simulink model "Balance"  (R2020a)
settings: Solver=FixedStepDiscrete  StartTime=0.0  StopTime=10.0  FixedStep=0.001  RelTol=1e-3
libraries: TIMERS_Lib x5, GPIO_Lib x4, USART_Lib x1, STM32_Config_Lib x1
settings Model: Creator=xiang  LastModifiedBy=Administrator
settings OptimizationCC: DefaultParameterBehavior=Inlined  EnhancedBackFolding=on  PassReuseOutputArgsAs=Individual arguments  ZeroExternalMemoryAtStartup=off  ZeroInternalMemoryAtStartup=off  OptimizeBlockOrder=speed  DifferentSizesBufferReuse=on  OptimizationCustomize=off  EfficientTunableParamExpr=on
settings DebuggingCC: MultiTaskDSMMsg=none  ParameterTunabilityLossMsg=error
settings HardwareCC: ProdBitPerPointer=32  ProdBitPerSizeT=32  ProdBitPerPtrDiffT=32  ProdLargestAtomicInteger=Long  ProdWordSize=32  ProdHWDeviceType=STM32CortexM
settings SFSimCC: SimCustomHeaderCode="#include \"myfile.h\""  SimUserSources="\"D:\\BMS\\CubeMx\\CubeMx_0804\\XSZ20210804\\myfile.c\""  MATLABDynamicMemAlloc=off
settings RTWCC: Description=stm32 (Embedded Target)  SystemTargetFile=stm32.tlc  TemplateMakefile=stm32.tmf  GenerateReport=on  RTWUseSimCustomCode=on  CustomHeaderCode="#include \"myfile.h\""  CustomSource="\"D:\\BMS\\CubeMx\\CubeMx_0804\\XSZ20210804\\myfile.c\""
settings CodeAppCC: ForceParamTrailComments=on  IgnoreCustomStorageClasses=off  MaxIdLength=64  OperatorAnnotations=on  SimulinkDataObjDesc=on  SFDataObjDesc=on  CustomSymbolStrType=$N$R$M  SimulinkBlockComments=off
settings STFCustomTargetCC: TargetLangStandard=C99 (ISO)  CodeReplacementLibrary=ARM CMSIS SIN COS  MultiwordLength=256  ParMdlRefBuildCompliant=on  IncludeMdlTerminateFcn=off  CombineOutputUpdateFcns=on  ERTCustomFileBanners=on  SupportContinuousTime=off  SupportNonInlinedSFcns=off  RemoveResetFunc=on  MATLABClassNameForMDSCustomization=Simulink.SoftwareTarget.ERTCustomization  SystemTargetFile=stm32.tlc
settings ERTTargetCC: TargetLangStandard=C99 (ISO)  CodeReplacementLibrary=ARM CMSIS SIN COS  CompOptLevelCompliant=off  ConcurrentExecutionCompliant=off  IncludeMdlTerminateFcn=off  ModelStepFunctionPrototypeControlCompliant=off  CPPClassGenCompliant=off  UseToolchainInfoCompliant=off  ExtModeStaticAllocSize=256  ExtModeMexFile=ext_serial_win32_comm  ExtModeMexArgs=0,1,115200,10  InlinedParameterPlacement=NonHierarchical  ERTSrcFileBannerTemplate=sourceFileTemplate.cgt  ERTHdrFileBannerTemplate=sourceFileTemplate.cgt  ERTDataSrcFileTemplate=sourceFileTemplate.cgt  ERTDataHdrFileTemplate=sourceFileTemplate.cgt  ERTCustomFileTemplate=customRoutineProcess.tlc

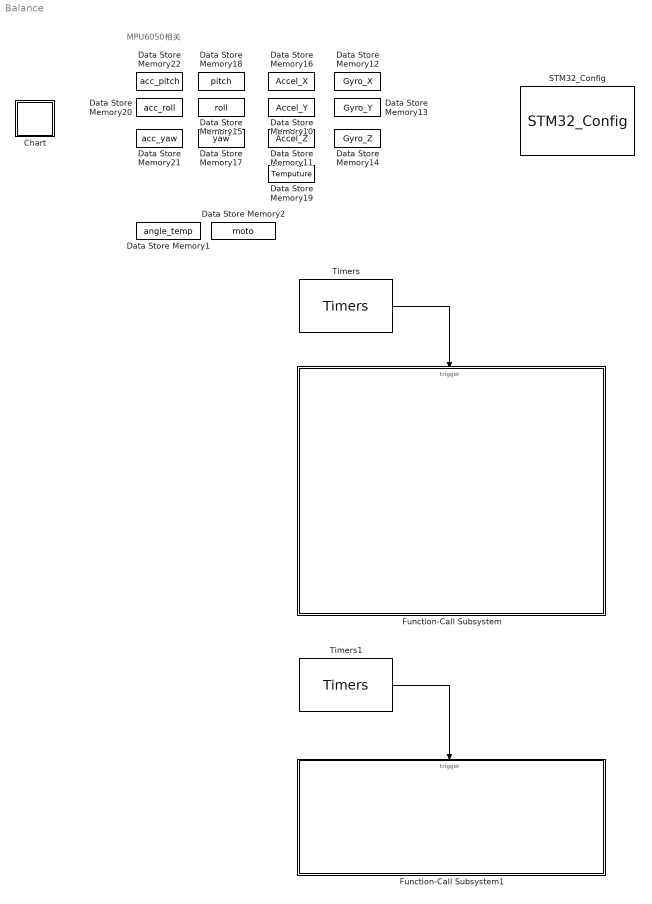
== system Balance ==
  note: MPU6050相关
  Chart : Stateflow chart  Priority=1  TreatAsAtomicUnit=on
  Data Store Memory1 : DataStoreMemory  DataStoreName=angle_temp  ReadBeforeWriteMsg=warning  WriteAfterWriteMsg=warning  WriteAfterReadMsg=warning  ShowAdditionalParam=off  OutDataTypeStr=single
      settings: RTWStateStorageClass=ExportedGlobal
  Data Store Memory10 : DataStoreMemory  DataStoreName=Accel_Y  ReadBeforeWriteMsg=warning  WriteAfterWriteMsg=warning  WriteAfterReadMsg=warning  ShowAdditionalParam=off  OutDataTypeStr=double
      settings: RTWStateStorageClass=ExportedGlobal
  Data Store Memory11 : DataStoreMemory  DataStoreName=Accel_Z  ReadBeforeWriteMsg=warning  WriteAfterWriteMsg=warning  WriteAfterReadMsg=warning  ShowAdditionalParam=off  OutDataTypeStr=double
      settings: RTWStateStorageClass=ExportedGlobal
  Data Store Memory12 : DataStoreMemory  DataStoreName=Gyro_X  ReadBeforeWriteMsg=warning  WriteAfterWriteMsg=warning  WriteAfterReadMsg=warning  ShowAdditionalParam=off  OutDataTypeStr=double
      settings: RTWStateStorageClass=ExportedGlobal
  Data Store Memory13 : DataStoreMemory  DataStoreName=Gyro_Y  ReadBeforeWriteMsg=warning  WriteAfterWriteMsg=warning  WriteAfterReadMsg=warning  ShowAdditionalParam=off  OutDataTypeStr=double
      settings: RTWStateStorageClass=ExportedGlobal
  Data Store Memory14 : DataStoreMemory  DataStoreName=Gyro_Z  ReadBeforeWriteMsg=warning  WriteAfterWriteMsg=warning  WriteAfterReadMsg=warning  ShowAdditionalParam=off  OutDataTypeStr=double
      settings: RTWStateStorageClass=ExportedGlobal
  Data Store Memory15 : DataStoreMemory  DataStoreName=roll  ReadBeforeWriteMsg=warning  WriteAfterWriteMsg=warning  WriteAfterReadMsg=warning  ShowAdditionalParam=off  OutDataTypeStr=double
      settings: RTWStateStorageClass=ExportedGlobal
  Data Store Memory16 : DataStoreMemory  DataStoreName=Accel_X  ReadBeforeWriteMsg=warning  WriteAfterWriteMsg=warning  WriteAfterReadMsg=warning  ShowAdditionalParam=off  OutDataTypeStr=double
      settings: RTWStateStorageClass=ExportedGlobal
  Data Store Memory17 : DataStoreMemory  DataStoreName=yaw  ReadBeforeWriteMsg=warning  WriteAfterWriteMsg=warning  WriteAfterReadMsg=warning  ShowAdditionalParam=off  OutDataTypeStr=double
      settings: RTWStateStorageClass=ExportedGlobal
  Data Store Memory18 : DataStoreMemory  DataStoreName=pitch  ReadBeforeWriteMsg=warning  WriteAfterWriteMsg=warning  WriteAfterReadMsg=warning  ShowAdditionalParam=off  OutDataTypeStr=double
      settings: RTWStateStorageClass=ExportedGlobal
  Data Store Memory19 : DataStoreMemory  DataStoreName=Temputure  ReadBeforeWriteMsg=warning  WriteAfterWriteMsg=warning  WriteAfterReadMsg=warning  ShowAdditionalParam=off  OutDataTypeStr=double
      settings: RTWStateStorageClass=ExportedGlobal
  Data Store Memory2 : DataStoreMemory  DataStoreName=moto  ReadBeforeWriteMsg=warning  WriteAfterWriteMsg=warning  WriteAfterReadMsg=warning  ShowAdditionalParam=off  OutDataTypeStr=double
      settings: RTWStateStorageClass=ExportedGlobal
  Data Store Memory20 : DataStoreMemory  DataStoreName=acc_roll  ReadBeforeWriteMsg=warning  WriteAfterWriteMsg=warning  WriteAfterReadMsg=warning  ShowAdditionalParam=off  OutDataTypeStr=double
      settings: RTWStateStorageClass=ExportedGlobal
  Data Store Memory21 : DataStoreMemory  DataStoreName=acc_yaw  ReadBeforeWriteMsg=warning  WriteAfterWriteMsg=warning  WriteAfterReadMsg=warning  ShowAdditionalParam=off  OutDataTypeStr=double
      settings: RTWStateStorageClass=ExportedGlobal
  Data Store Memory22 : DataStoreMemory  DataStoreName=acc_pitch  ReadBeforeWriteMsg=warning  WriteAfterWriteMsg=warning  WriteAfterReadMsg=warning  ShowAdditionalParam=off  OutDataTypeStr=double
      settings: RTWStateStorageClass=ExportedGlobal
  Function-Call Subsystem : Subsystem  TreatAsAtomicUnit=on
  Function-Call Subsystem1 : Subsystem  TreatAsAtomicUnit=on
  STM32_Config : STM32_Config_Lib/STM32_Config  Priority=0  Project_Path=.\  Config_File=XSZ20210804.ioc  MCU_Name=STM32F103VETx
      settings: SourceProductName=Target Support Package - STM32 Adapter
  Timers : TIMERS_Lib/Timers  currentTIM=TIM1  TIM_Name=TIM1  sysUsingTimer=off  TIM_APBClock=72000000  TIM_Set_Clk=off  TIM_Prescaler=7199  TIM_Clock=10000.00  Variable_frequency=off  TIM_Set_OutFreq=on  TIM_ARR=50  Output_frequency=200.00  Repetition_counter=0  TIM_Mode=Up  TIM_DMA=none  TIM_IRQ=off  TIM_IRQ_ONLY=on  TIM_UP=on  TIM_TRG=off  TIM_COM=off  TIM_BRK=off  NbTIM=3  CH1_enable=off  CH1N_enable=off  CH1_type=Unknown  CH1_DMA=off  CH1_int=off  CH1_edge=Rising  CH1_div=1  CH1_variable_duty=off  CH1_set_pulse=off  CH1_output_duty=0.00  CH1_pulse=0  CH2_enable=off  CH2N_enable=off  CH2_type=Unknown  CH2_DMA=off  CH2_int=off  CH2_edge=Rising  CH2_div=1  CH2_variable_duty=off  CH2_set_pulse=off  CH2_output_duty=0.00  CH2_pulse=0  CH3_enable=off  CH3N_enable=off  CH3_type=Unknown  CH3_DMA=off  CH3_int=off  CH3_edge=Rising  CH3_div=1  CH3_variable_duty=off  CH3_set_pulse=off  CH3_output_duty=0.00  CH3_pulse=0  CH4_enable=off  CH4N_enable=off  CH4_type=Unknown  CH4_DMA=off  CH4_int=off  CH4_edge=Rising  CH4_div=1  CH4_variable_duty=off  CH4_set_pulse=off  CH4_output_duty=0.00  CH4_pulse=0
      settings: SourceProductName=Target Support Package - STM32 Adapter
  Timers1 : TIMERS_Lib/Timers  currentTIM=TIM3  TIM_Name=TIM3  sysUsingTimer=off  TIM_APBClock=72000000  TIM_Set_Clk=off  TIM_Prescaler=7199  TIM_Clock=10000.00  Variable_frequency=off  TIM_Set_OutFreq=off  TIM_ARR=1000  Output_frequency=10.00  Repetition_counter=0  TIM_Mode=Up  TIM_DMA=none  TIM_IRQ=on  TIM_IRQ_ONLY=on  TIM_UP=on  TIM_TRG=off  TIM_COM=off  TIM_BRK=off  NbTIM=3  CH1_enable=off  CH1N_enable=off  CH1_type=Unknown  CH1_DMA=off  CH1_int=off  CH1_edge=Rising  CH1_div=1  CH1_variable_duty=off  CH1_set_pulse=off  CH1_output_duty=0.00  CH1_pulse=0  CH2_enable=off  CH2N_enable=off  CH2_type=Unknown  CH2_DMA=off  CH2_int=off  CH2_edge=Rising  CH2_div=1  CH2_variable_duty=off  CH2_set_pulse=off  CH2_output_duty=0.00  CH2_pulse=0  CH3_enable=off  CH3N_enable=off  CH3_type=Unknown  CH3_DMA=off  CH3_int=off  CH3_edge=Rising  CH3_div=1  CH3_variable_duty=off  CH3_set_pulse=off  CH3_output_duty=0.00  CH3_pulse=0  CH4_enable=off  CH4N_enable=off  CH4_type=Unknown  CH4_DMA=off  CH4_int=off  CH4_edge=Rising  CH4_div=1  CH4_variable_duty=off  CH4_set_pulse=off  CH4_output_duty=0.00  CH4_pulse=0
      settings: SourceProductName=Target Support Package - STM32 Adapter
  wires:
  Timers/1 -> Function-Call Subsystem/Trigger
  Timers1/1 -> Function-Call Subsystem1/Trigger

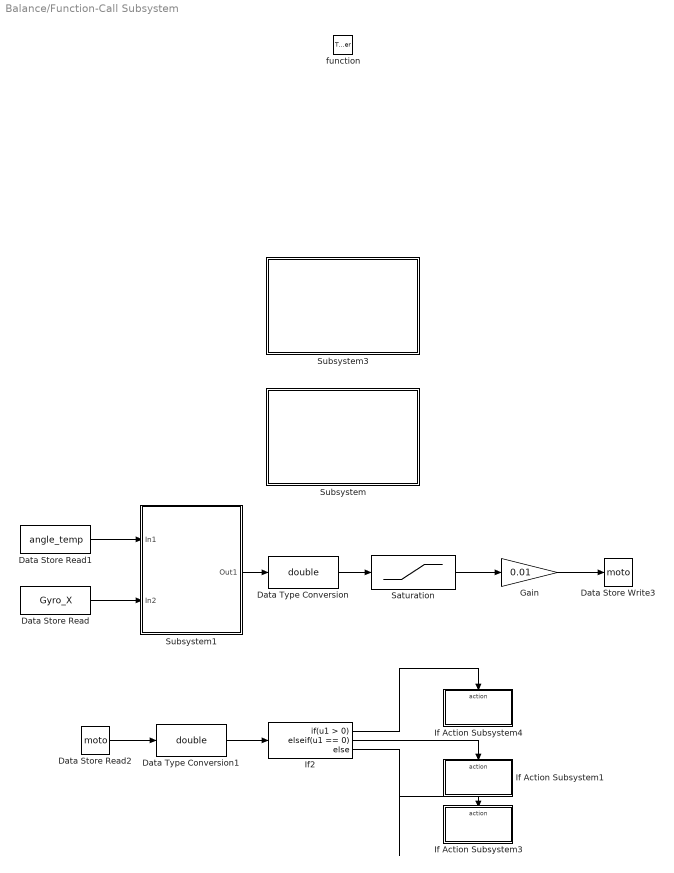
== system Balance/Function-Call Subsystem ==
  function : TriggerPort  TriggerType=function-call  VariantControl=Variant
  Data Store Read : DataStoreRead  DataStoreName=Gyro_X
  Data Store Read1 : DataStoreRead  DataStoreName=angle_temp
  Data Store Read2 : DataStoreRead  DataStoreName=moto
  Data Store Write3 : DataStoreWrite  DataStoreName=moto
  Data Type Conversion : DataTypeConversion  OutDataTypeStr=double
  Data Type Conversion1 : DataTypeConversion  OutDataTypeStr=double
  Gain : Gain  Gain=0.01
  If Action Subsystem1 : Subsystem  TreatAsAtomicUnit=on
  If Action Subsystem3 : Subsystem  TreatAsAtomicUnit=on
  If Action Subsystem4 : Subsystem  TreatAsAtomicUnit=on
  If2 : If  ElseIfExpressions=u1 == 0
  Saturation : Saturate  UpperLimit=1000  LowerLimit=-1000
  Subsystem : Subsystem
  Subsystem1 : Subsystem  Priority=1
  Subsystem3 : Subsystem  Priority=2
  wires:
  If2/1 -> If Action Subsystem4/Action
  If2/2 -> If Action Subsystem1/Action
  If2/3 -> If Action Subsystem3/Action
  Data Store Read1/1 -> Subsystem1/1(In1)
  Data Store Read/1 -> Subsystem1/2(In2)
  Saturation/1 -> Gain/1
  Subsystem1/1(Out1) -> Data Type Conversion/1
  Data Type Conversion/1 -> Saturation/1
  Gain/1 -> Data Store Write3/1
  Data Store Read2/1 -> Data Type Conversion1/1
  Data Type Conversion1/1 -> If2/1

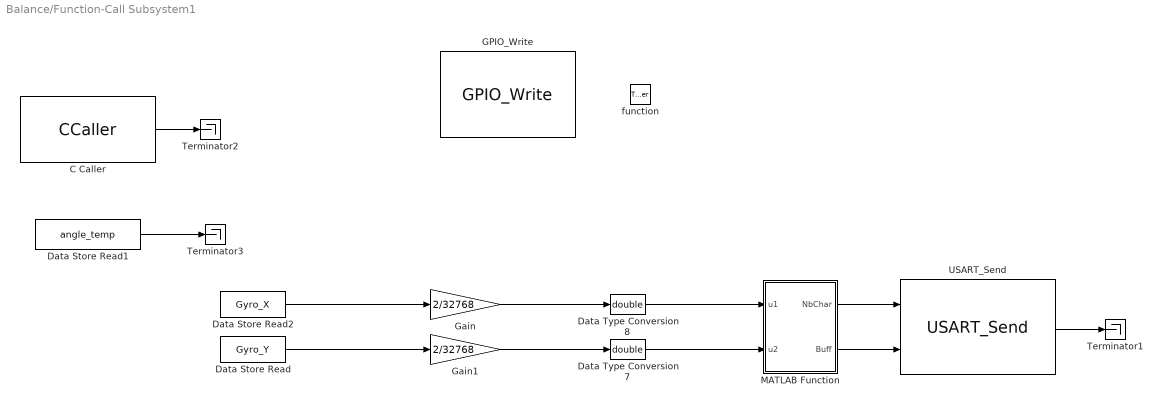
== system Balance/Function-Call Subsystem1 ==
  function : TriggerPort  TriggerType=function-call  VariantControl=Variant
  C Caller : CCaller  FunctionName=Read_Temperature  PortSpecificationStruct="%)30     .    & (   8    (     @         %    \"     $    !     0         %  0 \"0    $    _    07)G3F%M90  4&]R=$YA;64 4V-O<&4     26YD97@     5'EP90      4VEZ90      27-';&]B86P   X    P    !@    @    $          4    (     0    ,    !         !   P!O=70 #@   #     &    \"     0         !0    @    !     P    $         $  # &]U=  .    .     8    (    !          %    \"     $    &     0         0    !@   $]U='!U=   #@   #@    &    \"     8         !0    @    !     0    $         \"0    @               X    X    !@    @    $          4    (     0    4    !         !     %    :6YT,S(    .    ,     8    (    !          %    \"     $    !     0         0  $ ,0    X    P    !@    @    ) @        4    (     0    $    !          (  0"
  Data Store Read : DataStoreRead  DataStoreName=Gyro_Y
  Data Store Read1 : DataStoreRead  DataStoreName=angle_temp
  Data Store Read2 : DataStoreRead  DataStoreName=Gyro_X
  Data Type Conversion7 : DataTypeConversion  OutDataTypeStr=double
  Data Type Conversion8 : DataTypeConversion  OutDataTypeStr=double
  GPIO_Write : GPIO_Lib/GPIO_Write  Port_name=GPIOB  Pin0=on  Toggle_Pin0=on  Pin1=off  Toggle_Pin1=off  Pin2=off  Toggle_Pin2=off  Pin3=off  Toggle_Pin3=off  Pin4=off  Toggle_Pin4=off  Pin5=off  Toggle_Pin5=off  Pin6=off  Toggle_Pin6=off  Pin7=off  Toggle_Pin7=off  Pin8=off  Toggle_Pin8=off  Pin9=off  Toggle_Pin9=off  Pin10=off  Toggle_Pin10=off  Pin11=off  Toggle_Pin11=off  Pin12=off  Toggle_Pin12=off  Pin13=off  Toggle_Pin13=off  Pin14=off  Toggle_Pin14=off  Pin15=off  Toggle_Pin15=off  PinList="GPIOA4  5GPIOB0"
      settings: SourceProductName=Target Support Package - STM32 Adapter
  Gain : Gain  Gain=2/32768
  Gain1 : Gain  Gain=2/32768
  MATLAB Function : MATLAB Function  TreatAsAtomicUnit=on
  Terminator1 : Terminator
  Terminator2 : Terminator
  Terminator3 : Terminator
  USART_Send : USART_Lib/USART_Send  USART_name=USART1  Buff_size=500  nbUsart=1  usartMode=Asynchronous  usartDma_Rx=off  usartDma_Tx=off  usartIt=off
      settings: SourceProductName=Target Support Package - STM32 Adapter
  wires:
  Data Type Conversion8/1 -> MATLAB Function/1(u1)
  Data Type Conversion7/1 -> MATLAB Function/2(u2)
  MATLAB Function/2(Buff) -> USART_Send/2
  USART_Send/1 -> Terminator1/1
  MATLAB Function/1(NbChar) -> USART_Send/1
  C Caller/1 -> Terminator2/1
  Data Store Read1/1 -> Terminator3/1
  Data Store Read2/1 -> Gain/1
  Data Store Read/1 -> Gain1/1
  Gain/1 -> Data Type Conversion8/1
  Gain1/1 -> Data Type Conversion7/1

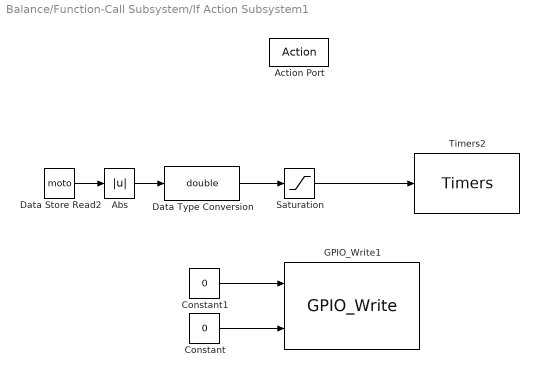
== system Balance/Function-Call Subsystem/If Action Subsystem1 ==
  Action Port : ActionPort  ActionPortLabel=elseif(u1 == 0)
  Abs : Abs
  Constant : Constant  Value=0
  Constant1 : Constant  Value=0
  Data Store Read2 : DataStoreRead  DataStoreName=moto
  Data Type Conversion : DataTypeConversion  OutDataTypeStr=double
  GPIO_Write1 : GPIO_Lib/GPIO_Write  Port_name=GPIOA  Pin0=off  Toggle_Pin0=off  Pin1=off  Toggle_Pin1=off  Pin2=off  Toggle_Pin2=off  Pin3=off  Toggle_Pin3=off  Pin4=on  Toggle_Pin4=off  Pin5=on  Toggle_Pin5=off  Pin6=off  Toggle_Pin6=off  Pin7=off  Toggle_Pin7=off  Pin8=off  Toggle_Pin8=off  Pin9=off  Toggle_Pin9=off  Pin10=off  Toggle_Pin10=off  Pin11=off  Toggle_Pin11=off  Pin12=off  Toggle_Pin12=off  Pin13=off  Toggle_Pin13=off  Pin14=off  Toggle_Pin14=off  Pin15=off  Toggle_Pin15=off  PinList="GPIOA4  5GPIOB0"
      settings: SourceProductName=Target Support Package - STM32 Adapter
  Saturation : Saturate  UpperLimit=100  LowerLimit=0
  Timers2 : TIMERS_Lib/Timers  currentTIM=TIM2  TIM_Name=TIM2  sysUsingTimer=off  TIM_APBClock=72000000  TIM_Set_Clk=off  TIM_Prescaler=71  TIM_Clock=1000000.00  Variable_frequency=off  TIM_Set_OutFreq=off  TIM_ARR=1000  Output_frequency=1000.00  Repetition_counter=0  TIM_Mode=Up  TIM_DMA=none  TIM_IRQ=off  TIM_IRQ_ONLY=off  TIM_UP=off  TIM_TRG=off  TIM_COM=off  TIM_BRK=off  NbTIM=3  CH1_enable=off  CH1N_enable=off  CH1_type=Unknown  CH1_DMA=off  CH1_int=off  CH1_edge=Rising  CH1_div=1  CH1_variable_duty=off  CH1_set_pulse=off  CH1_output_duty=0.00  CH1_pulse=0  CH2_enable=off  CH2N_enable=off  CH2_type=Unknown  CH2_DMA=off  CH2_int=off  CH2_edge=Rising  CH2_div=1  CH2_variable_duty=off  CH2_set_pulse=off  CH2_output_duty=0.00  CH2_pulse=0  CH3_enable=on  CH3N_enable=off  CH3_type=Output_PWM  CH3_DMA=off  CH3_int=off  CH3_edge=Rising  CH3_div=1  CH3_variable_duty=on  CH3_set_pulse=on  CH3_output_duty=80.00  CH3_pulse=800  CH4_enable=off  CH4N_enable=off  CH4_type=Unknown  CH4_DMA=off  CH4_int=off  CH4_edge=Rising  CH4_div=1  CH4_variable_duty=off  CH4_set_pulse=off  CH4_output_duty=0.00  CH4_pulse=0
      settings: SourceProductName=Target Support Package - STM32 Adapter
  wires:
  Constant1/1 -> GPIO_Write1/1
  Constant/1 -> GPIO_Write1/2
  Saturation/1 -> Timers2/1
  Data Type Conversion/1 -> Saturation/1
  Data Store Read2/1 -> Abs/1
  Abs/1 -> Data Type Conversion/1

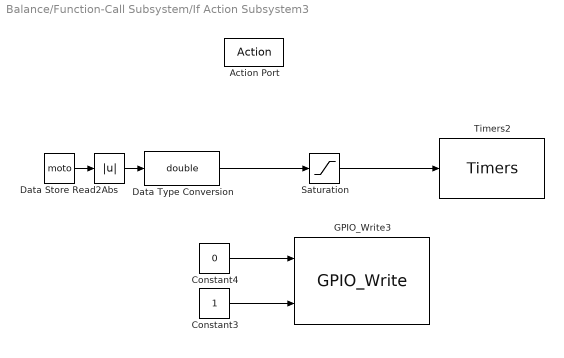
== system Balance/Function-Call Subsystem/If Action Subsystem3 ==
  Action Port : ActionPort  ActionPortLabel=else
  Abs : Abs
  Constant3 : Constant
  Constant4 : Constant  Value=0
  Data Store Read2 : DataStoreRead  DataStoreName=moto
  Data Type Conversion : DataTypeConversion  OutDataTypeStr=double
  GPIO_Write3 : GPIO_Lib/GPIO_Write  Port_name=GPIOA  Pin0=off  Toggle_Pin0=off  Pin1=off  Toggle_Pin1=off  Pin2=off  Toggle_Pin2=off  Pin3=off  Toggle_Pin3=off  Pin4=on  Toggle_Pin4=off  Pin5=on  Toggle_Pin5=off  Pin6=off  Toggle_Pin6=off  Pin7=off  Toggle_Pin7=off  Pin8=off  Toggle_Pin8=off  Pin9=off  Toggle_Pin9=off  Pin10=off  Toggle_Pin10=off  Pin11=off  Toggle_Pin11=off  Pin12=off  Toggle_Pin12=off  Pin13=off  Toggle_Pin13=off  Pin14=off  Toggle_Pin14=off  Pin15=off  Toggle_Pin15=off  PinList="GPIOA4  5GPIOB0"
      settings: SourceProductName=Target Support Package - STM32 Adapter
  Saturation : Saturate  UpperLimit=100  LowerLimit=0
  Timers2 : TIMERS_Lib/Timers  currentTIM=TIM2  TIM_Name=TIM2  sysUsingTimer=off  TIM_APBClock=72000000  TIM_Set_Clk=off  TIM_Prescaler=71  TIM_Clock=1000000.00  Variable_frequency=off  TIM_Set_OutFreq=off  TIM_ARR=1000  Output_frequency=1000.00  Repetition_counter=0  TIM_Mode=Up  TIM_DMA=none  TIM_IRQ=off  TIM_IRQ_ONLY=off  TIM_UP=off  TIM_TRG=off  TIM_COM=off  TIM_BRK=off  NbTIM=3  CH1_enable=off  CH1N_enable=off  CH1_type=Unknown  CH1_DMA=off  CH1_int=off  CH1_edge=Rising  CH1_div=1  CH1_variable_duty=off  CH1_set_pulse=off  CH1_output_duty=0.00  CH1_pulse=0  CH2_enable=off  CH2N_enable=off  CH2_type=Unknown  CH2_DMA=off  CH2_int=off  CH2_edge=Rising  CH2_div=1  CH2_variable_duty=off  CH2_set_pulse=off  CH2_output_duty=0.00  CH2_pulse=0  CH3_enable=on  CH3N_enable=off  CH3_type=Output_PWM  CH3_DMA=off  CH3_int=off  CH3_edge=Rising  CH3_div=1  CH3_variable_duty=on  CH3_set_pulse=on  CH3_output_duty=80.00  CH3_pulse=800  CH4_enable=off  CH4N_enable=off  CH4_type=Unknown  CH4_DMA=off  CH4_int=off  CH4_edge=Rising  CH4_div=1  CH4_variable_duty=off  CH4_set_pulse=off  CH4_output_duty=0.00  CH4_pulse=0
      settings: SourceProductName=Target Support Package - STM32 Adapter
  wires:
  Constant4/1 -> GPIO_Write3/1
  Constant3/1 -> GPIO_Write3/2
  Saturation/1 -> Timers2/1
  Data Type Conversion/1 -> Saturation/1
  Data Store Read2/1 -> Abs/1
  Abs/1 -> Data Type Conversion/1

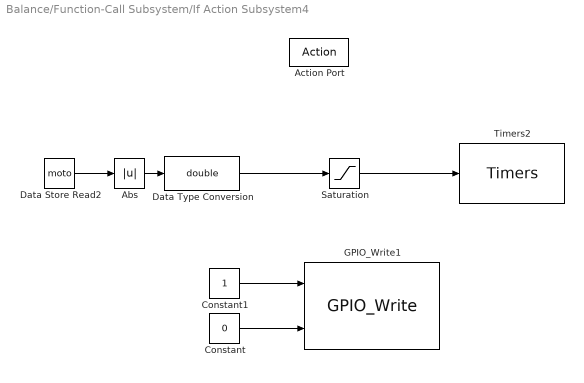
== system Balance/Function-Call Subsystem/If Action Subsystem4 ==
  Action Port : ActionPort  ActionPortLabel=if(u1 > 0)
  Abs : Abs
  Constant : Constant  Value=0
  Constant1 : Constant
  Data Store Read2 : DataStoreRead  DataStoreName=moto
  Data Type Conversion : DataTypeConversion  OutDataTypeStr=double
  GPIO_Write1 : GPIO_Lib/GPIO_Write  Port_name=GPIOA  Pin0=off  Toggle_Pin0=off  Pin1=off  Toggle_Pin1=off  Pin2=off  Toggle_Pin2=off  Pin3=off  Toggle_Pin3=off  Pin4=on  Toggle_Pin4=off  Pin5=on  Toggle_Pin5=off  Pin6=off  Toggle_Pin6=off  Pin7=off  Toggle_Pin7=off  Pin8=off  Toggle_Pin8=off  Pin9=off  Toggle_Pin9=off  Pin10=off  Toggle_Pin10=off  Pin11=off  Toggle_Pin11=off  Pin12=off  Toggle_Pin12=off  Pin13=off  Toggle_Pin13=off  Pin14=off  Toggle_Pin14=off  Pin15=off  Toggle_Pin15=off  PinList="GPIOA4  5GPIOB0"
      settings: SourceProductName=Target Support Package - STM32 Adapter
  Saturation : Saturate  UpperLimit=100  LowerLimit=0
  Timers2 : TIMERS_Lib/Timers  currentTIM=TIM2  TIM_Name=TIM2  sysUsingTimer=off  TIM_APBClock=72000000  TIM_Set_Clk=off  TIM_Prescaler=71  TIM_Clock=1000000.00  Variable_frequency=off  TIM_Set_OutFreq=off  TIM_ARR=1000  Output_frequency=1000.00  Repetition_counter=0  TIM_Mode=Up  TIM_DMA=none  TIM_IRQ=off  TIM_IRQ_ONLY=off  TIM_UP=off  TIM_TRG=off  TIM_COM=off  TIM_BRK=off  NbTIM=3  CH1_enable=off  CH1N_enable=off  CH1_type=Unknown  CH1_DMA=off  CH1_int=off  CH1_edge=Rising  CH1_div=1  CH1_variable_duty=off  CH1_set_pulse=off  CH1_output_duty=0.00  CH1_pulse=0  CH2_enable=off  CH2N_enable=off  CH2_type=Unknown  CH2_DMA=off  CH2_int=off  CH2_edge=Rising  CH2_div=1  CH2_variable_duty=off  CH2_set_pulse=off  CH2_output_duty=0.00  CH2_pulse=0  CH3_enable=on  CH3N_enable=off  CH3_type=Output_PWM  CH3_DMA=off  CH3_int=off  CH3_edge=Rising  CH3_div=1  CH3_variable_duty=on  CH3_set_pulse=on  CH3_output_duty=80.00  CH3_pulse=800  CH4_enable=off  CH4N_enable=off  CH4_type=Unknown  CH4_DMA=off  CH4_int=off  CH4_edge=Rising  CH4_div=1  CH4_variable_duty=off  CH4_set_pulse=off  CH4_output_duty=0.00  CH4_pulse=0
      settings: SourceProductName=Target Support Package - STM32 Adapter
  wires:
  Constant/1 -> GPIO_Write1/2
  Constant1/1 -> GPIO_Write1/1
  Saturation/1 -> Timers2/1
  Data Type Conversion/1 -> Saturation/1
  Data Store Read2/1 -> Abs/1
  Abs/1 -> Data Type Conversion/1

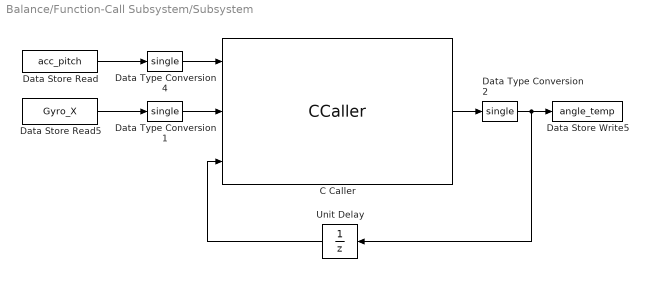
== system Balance/Function-Call Subsystem/Subsystem ==
  C Caller : CCaller  FunctionName=Kalman_Filter  PortSpecificationStruct="%)30     .    & <   8    (     @         %    \"     0    !     0         %  0 \"0    $    _    07)G3F%M90  4&]R=$YA;64 4V-O<&4     26YD97@     5'EP90      4VEZ90      27-';&]B86P   X    P    !@    @    $          4    (     0    ,    !         !   P!O=70 #@   #     &    \"     0         !0    @    !     P    $         $  # &]U=  .    .     8    (    !          %    \"     $    &     0         0   ...(+2061 chars)"
  Data Store Read : DataStoreRead  DataStoreName=acc_pitch
  Data Store Read5 : DataStoreRead  DataStoreName=Gyro_X
  Data Store Write5 : DataStoreWrite  DataStoreName=angle_temp
  Data Type Conversion1 : DataTypeConversion  OutDataTypeStr=single
  Data Type Conversion2 : DataTypeConversion  OutDataTypeStr=single
  Data Type Conversion4 : DataTypeConversion  OutDataTypeStr=single
  Unit Delay : UnitDelay  SampleTime=-1  HasFrameUpgradeWarning=on
  wires:
  C Caller/1 -> Data Type Conversion2/1
  Data Store Read/1 -> Data Type Conversion4/1
  Data Store Read5/1 -> Data Type Conversion1/1
  Data Type Conversion1/1 -> C Caller/2
  Data Type Conversion4/1 -> C Caller/1
  Data Type Conversion2/1 -> Unit Delay/1, Data Store Write5/1
  Unit Delay/1 -> C Caller/3

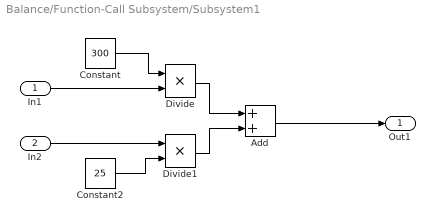
== system Balance/Function-Call Subsystem/Subsystem1 ==
  In1 : Inport
  In2 : Inport  Port=2
  Add : Sum
  Constant : Constant  Value=300
  Constant2 : Constant  Value=25
  Divide : Product  Inputs=**
  Divide1 : Product  Inputs=**
  Out1 : Outport  VectorParamsAs1DForOutWhenUnconnected=off
  wires:
  Divide1/1 -> Add/2
  Constant/1 -> Divide/1
  Constant2/1 -> Divide1/2
  Add/1 -> Out1/1
  Divide/1 -> Add/1
  In1/1 -> Divide/2
  In2/1 -> Divide1/1

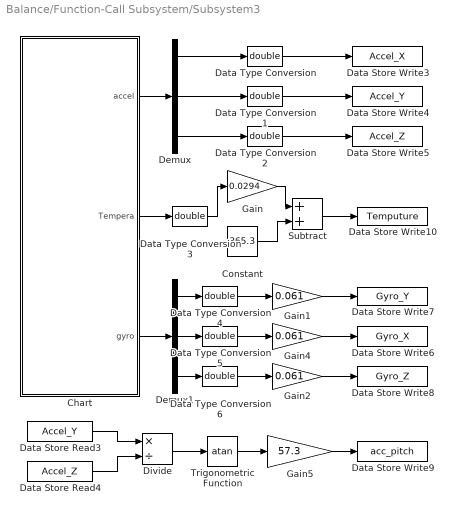
== system Balance/Function-Call Subsystem/Subsystem3 ==
  Chart : Stateflow chart  TreatAsAtomicUnit=on
  Constant : Constant  Value=365.3  OutDataTypeStr=double
  Data Store Read3 : DataStoreRead  DataStoreName=Accel_Y
  Data Store Read4 : DataStoreRead  DataStoreName=Accel_Z
  Data Store Write10 : DataStoreWrite  DataStoreName=Temputure
  Data Store Write3 : DataStoreWrite  DataStoreName=Accel_X
  Data Store Write4 : DataStoreWrite  DataStoreName=Accel_Y
  Data Store Write5 : DataStoreWrite  DataStoreName=Accel_Z
  Data Store Write6 : DataStoreWrite  DataStoreName=Gyro_X
  Data Store Write7 : DataStoreWrite  DataStoreName=Gyro_Y
  Data Store Write8 : DataStoreWrite  DataStoreName=Gyro_Z
  Data Store Write9 : DataStoreWrite  DataStoreName=acc_pitch
  Data Type Conversion{,1..6} (7 alike) : DataTypeConversion  OutDataTypeStr=double
  Demux : Demux  Outputs=3
  Demux1 : Demux  Outputs=3
  Divide : Product  Inputs=*/
  Gain : Gain  Gain=0.0294  OutDataTypeStr=double
  Gain1 : Gain  Gain=0.061  OutDataTypeStr=double
  Gain2 : Gain  Gain=0.061  OutDataTypeStr=double
  Gain4 : Gain  Gain=0.061  OutDataTypeStr=double
  Gain5 : Gain  Gain=57.3  OutDataTypeStr=double
  Subtract : Sum  OutDataTypeStr=double
  Trigonometric Function : Trigonometry  Operator=atan
  wires:
  Demux/2 -> Data Type Conversion1/1
  Demux/1 -> Data Type Conversion/1
  Demux/3 -> Data Type Conversion2/1
  Demux1/2 -> Data Type Conversion5/1
  Demux1/3 -> Data Type Conversion6/1
  Demux1/1 -> Data Type Conversion4/1
  Chart/3(gyro) -> Demux1/1
  Chart/1(accel) -> Demux/1
  Gain/1 -> Subtract/1
  Constant/1 -> Subtract/2
  Subtract/1 -> Data Store Write10/1
  Gain1/1 -> Data Store Write7/1
  Gain4/1 -> Data Store Write6/1
  Gain2/1 -> Data Store Write8/1
  Data Type Conversion/1 -> Data Store Write3/1
  Data Type Conversion1/1 -> Data Store Write4/1
  Data Type Conversion2/1 -> Data Store Write5/1
  Chart/2(Tempera) -> Data Type Conversion3/1
  Data Type Conversion3/1 -> Gain/1
  Data Type Conversion4/1 -> Gain1/1
  Data Type Conversion6/1 -> Gain2/1
  Data Type Conversion5/1 -> Gain4/1
  Data Store Read4/1 -> Divide/2
  Data Store Read3/1 -> Divide/1
  Divide/1 -> Trigonometric Function/1
  Gain5/1 -> Data Store Write9/1
  Trigonometric Function/1 -> Gain5/1

== stateflow chart Balance/Function-Call Subsystem/Subsystem3/Chart ==
  (default) -> (junction 1)
  (junction 1) -> (junction 3) : {MPU6050ReadDATA(accel,Tempera,gyro);}
  data: accel output int16 size=3; Tempera output int16 size=1; gyro output int16 size=3

== stateflow chart Balance/Chart ==
  (default) -> (junction 51) : % i
  (junction 51) -> (junction 52) [order 1] : [i<1]
  (junction 51) -> (junction 53) [order 2] : [i>=1]
  (junction 52) -> (junction 54) : {IIC_Init();MPU6050_initialize();i = i + 1;}
  (junction 54) -> (junction 53)
  (junction 53) -> (junction 55)
  data: i local double

== matlab function Balance/Function-Call Subsystem1/MATLAB Function ==
  data: u1 input; NbChar output; Buff output; u2 input
function [NbChar, Buff] = convert(u1,u2)
if coder.target('Sfun')
% Executing in MATLAB, Buff is null
Buff = uint32(0);
NbChar = uint16(0);
else
% Executing in the generated code. 
%buffer is an array of 15 unsigned char
% buffer = zeros(1,32,'uint8');
% %Generate C code using sprintf to write input value as float in buffer
% coder.ceval('sprintf',coder.wref(buffer),['u1= %5.0f,u2= %5.0f',0],u1,u2);
% y = [buffer(1:22),13,10,0];
% %Call getBuffPtr extern C function to get pointer address of y buffer 
% Buff = coder.ceval('getBuffPtr',coder.ref(y));
% NbChar = uint16(size(y,2));

% Executing in the generated code.
string = char(zeros(1,23));
stringSize = uint16(size(string,2));
stringFormat = char(['u1= %5.2f,u2= %5.2f',13,10,0]);
coder.ceval('snprintf',coder.wref(string),stringSize,coder.rref(stringFormat),u1,u2);
Buff = coder.ceval('getBuffPtr',coder.rref(string));
NbChar = stringSize;

end
end
